simulink model "MPCFULLMODEL"  (R2022b)
settings: Solver=VariableStepAuto  StartTime=0.0  StopTime=Ts  RelTol=1e-3
values from neighbouring files (symbols this model uses):
  plantSwitch = i    [setT.m]
libraries: cstblocks x1, mpclib x1, simulink x1
settings Model: Creator=wvx67826  LastModifiedBy=wvx67826
settings SolverCC: ZeroCrossControl=EnableAll  AutoInsertRateTranBlk=on

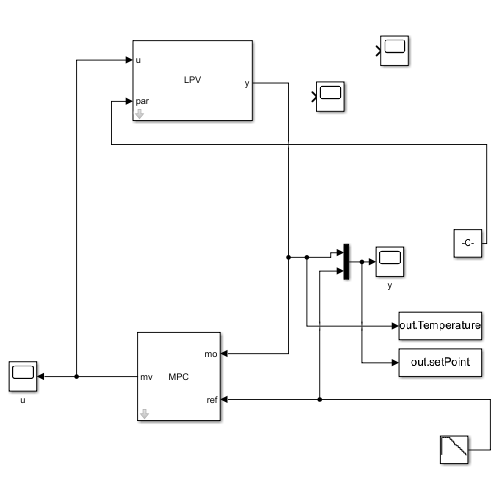
[thumbnail: Simulink's stored preview of the top-level diagram]
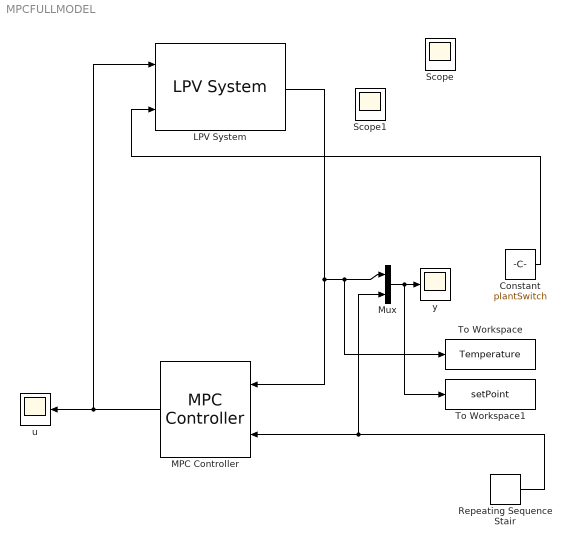
== system MPCFULLMODEL ==
  Constant : Constant  Value=plantSwitch
  LPV System : cstblocks/Linear Parameter Varying/LPV System  sys=sys  x0=0  uOffset=0  yOffset=0  xOffset=0  opEquilOption=off  dxOffset=0  sysFixedOption=Use the first model in state-space array  sysFixed=[]  AFixed=false  BFixed=false  CFixed=false  DFixed=false  uDelayFixed=false  yDelayFixed=false  iDelayFixed=false  IMethod=Nearest  EMethod=Clip  IndexSearch=Linear search  IndexBegin=on  OutputX=off  OutputXdot=off  OutputLTI=off  OutputOP=off  DataType=double  SimMode=Interpreted execution  InitBufferSize=1024  FixedBuffer=off
  MPC Controller : mpclib/MPC Controller  SCDEnableBlockLinearizationSpecification=on  mpcobj=mpcsss250400  is_multiple=0  enable_value=0  return_u0=off  updateMPCinCallerWorkspace=on  md_inport=off  mv_inport=off  uref_inport=off  return_cost=off  return_mvseq=off  return_qpstatus=off  return_xseq=off  return_state=off  return_ovseq=off  state_inport=off  umin_inport=off  umax_inport=off  ymin_inport=off  ymax_inport=off  cc_inport=off  ywt_inport=off  uwt_inport=off  duwt_inport=off  rhoeps_inport=off  pm_inport=off  MaximumP=10  HorizonChoice=FixedHorizon  n_ts=5  n_p=12  n_mv=1  n_md=0  n_ud=0  n_mo=1  n_uo=0  BlockDataType=double  SampleTimeInherited=off  switch_inport=off
  Mux : Mux  Inputs=2
  Repeating Sequence Stair : simulink/Sources/Repeating Sequence Stair  OutValues=tset  tsamp=stepwait  OutMin=[]  OutMax=[]  OutDataTypeStr=double  OutputDataTypeScalingMode=double  OutDataType=fixdt(0,8)  ConRadixGroup=Best Precision: Vector-wise  OutScaling=2^-12
  Scope : Scope
  Scope1 : Scope
  To Workspace : ToWorkspace  VariableName=Temperature  SampleTime=-1
  To Workspace1 : ToWorkspace  VariableName=setPoint  SampleTime=-1
  u : Scope
  y : Scope
  wires:
  Constant/1 -> LPV System/2
  Repeating Sequence Stair/1 -> Mux/2, MPC Controller/2
  Mux/1 -> To Workspace1/1, y/1
  MPC Controller/1 -> LPV System/1, u/1
  LPV System/1 -> To Workspace/1, Mux/1, MPC Controller/1
